simulink model "UnitTest_InitialConditionMng"  (Simulink 8.1)
settings: Solver=ode45  StartTime=0.0  StopTime=10.0  RelTol=1e-3
values from neighbouring files (symbols this model uses):
  Ts = 100E-6    (= 0.0001)    [RELAY_TEST_init.m]
libraries: relay_tripOutMng_lib x1
settings Model: Creator=re25624  LastModifiedBy=re25624
settings DataIOCC: SignalLoggingSaveFormat=Dataset
settings OptimizationCC: ExpressionDepthLimit=128
settings DebuggingCC: FcnCallInpInsideContextMsg=EnableAllAsError
settings GRTTargetCC: CombineOutputUpdateFcns=on  GRTInterface=off

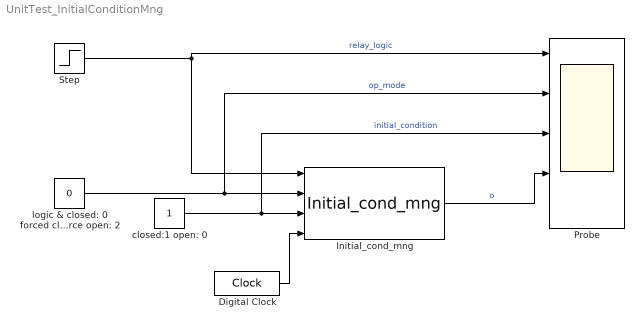
== system UnitTest_InitialConditionMng ==
  Digital Clock : DigitalClock  SampleTime=Ts
  Initial_cond_mng : relay_tripOutMng_lib/Initial_cond_mng
  Probe : Scope  NumInputPorts=5
      settings: TimeRange=10  YMin=0~-1~0~0~-5  YMax=1~1~2~2~5
  Step : Step  Time=5  Before=1  After=0  SampleTime=Ts
  closed:1 open: 0 : Constant
  logic & closed: 0 forced closed: 1 force open: 2 : Constant  Value=0
  wires:
  Step/1 -> Initial_cond_mng/1, Probe/1  "relay_logic"
  logic & closed: 0 forced closed: 1 force open: 2/1 -> Probe/2, Initial_cond_mng/2  "op_mode"
  closed:1 open: 0/1 -> Probe/3, Initial_cond_mng/3  "initial_condition"
  Initial_cond_mng/1 -> Probe/4  "o"
  Digital Clock/1 -> Initial_cond_mng/4
